simulink subsystem "MPC8_nlpsol"  (R2022b)
settings: Solver=VariableStepAuto  StartTime=0.0  StopTime=10.0  RelTol=1e-3
undefined symbols (not defined in the file): param_global, param_jointspace_ct, param_MPC8, param_robot, param_traj_data, param_weight_init
settings Model: Creator=emu  LastModifiedBy=emu
settings OptimizationCC: ReuseModelBlockBuffer=on

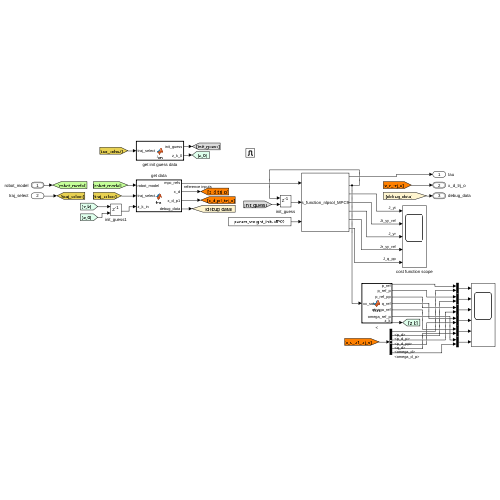
[thumbnail: Simulink's stored preview of the top-level diagram]
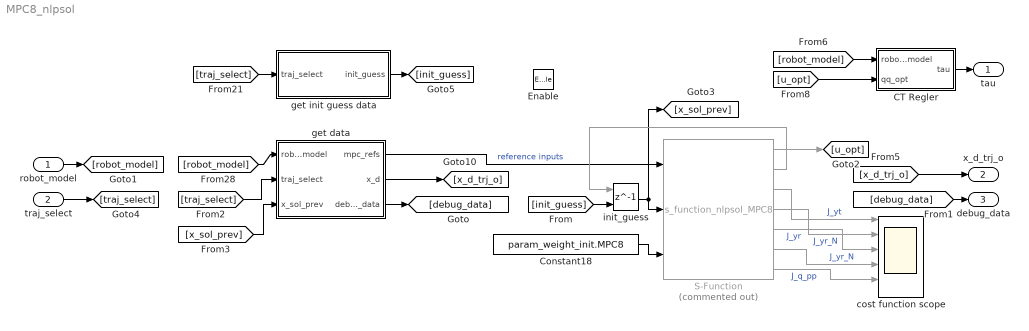
== system MPC8_nlpsol ==
  robot_model : Inport  OutDataTypeStr=Bus: robot_model
  traj_select : Inport  Port=2
  Enable : EnablePort
  CT Regler : MATLAB Function  TreatAsAtomicUnit=on
  Constant18 : Constant  Value=param_weight_init.MPC8  VectorParams1D=off
  S-Function : S-Function  Commented=on  FunctionName=s_function_nlpsol_MPC8  Parameters='s_functions/ur5e_6dof/MPC8.casadi', 'MPC8'  SFunctionModules='MPC8'  SFunctionDeploymentMode=off  EnableBusSupport=off
  cost function scope : Scope  NumInputPorts=6
  get data : MATLAB Function  TreatAsAtomicUnit=on
  get init guess data : MATLAB Function  TreatAsAtomicUnit=on
  init_guess : Delay  DelayLength=1  InitialConditionSource=Input port  InitialCondition=1
      settings: InputPortMap=u0,p4
  tau : Outport
  x_d_trj_o : Outport  Port=2  OutDataTypeStr=Bus: x_d
  debug_data : Outport  Port=3  OutDataTypeStr=Bus: debug_data_bus
  wires:
  S-Function/1 -> [u_opt]
  CT Regler/1(tau) -> tau/1
  [u_opt] -> CT Regler/2(qq_opt)
  [robot_model] -> CT Regler/1(robot_model)
  [x_d_trj_o] -> x_d_trj_o/1
  S-Function/3 -> cost function scope/1  "J_yt"
  robot_model/1 -> [robot_model]
  get data/2(x_d) -> [x_d_trj_o]
  S-Function/7 -> cost function scope/5  "J_q_pp"
  [traj_select] -> get init guess data/1(traj_select)
  get data/1(mpc_refs) -> S-Function/1  "reference inputs"
  [robot_model] -> get data/1(robot_model)
  get init guess data/1(init_guess) -> [init_guess]
  traj_select/1 -> [traj_select]
  init_guess/1 -> [x_sol_prev], S-Function/2
  [traj_select] -> get data/2(traj_select)
  [init_guess] -> init_guess/2
  S-Function/5 -> cost function scope/3  "J_yr"
  get data/3(debug_data) -> [debug_data]
  [debug_data] -> debug_data/1
  Constant18/1 -> S-Function/3
  S-Function/2 -> init_guess/1
  S-Function/4 -> cost function scope/2  "J_yr_N"
  S-Function/6 -> cost function scope/4  "J_yr_N"
  ? -> cost function scope/6  "J_du"
  [x_sol_prev] -> get data/3(x_sol_prev)

== matlab function MPC8_nlpsol/CT Regler ==
  data: robot_model input Bus: robot_model; tau output; qq_opt input; param_robot parameter; param_jointspace_ct parameter; param_global parameter
function tau = fcn(robot_model, qq_opt, param_robot, param_jointspace_ct, param_global)

n = param_robot.n_DOF;

if size(qq_opt, 2) ~= 0 && size(qq_opt, 1) ~= 1
    Ta = param_global.Ta;
    q = robot_model.q;      % generalized coordinates
    q_p = robot_model.q_p;  % time derivative of generalized coordinates
    
    q_d = qq_opt(1:n);
    q_d_p = qq_opt(n+1:2*n);
    q_d_pp = qq_opt(2*n+1:end);
    
    %q_d = q_d_0 + Ta*q_d_p_0;
    %q_d_p = q_d_p_0 + Ta*q_d_pp_0;
    %q_d_pp = q_d_pp_0;

    M = robot_model.M;      % inertia matrix
    C_rnea = robot_model.C_rnea; % C_rnea(q, q_p) = C(q, q_p)q_p + g(q) = n(q, q_p)
    
    e = q - q_d;
    e_p = q_p - q_d_p;
    
    K_D_q = param_jointspace_ct.MPC8.K_D_q;
    K_P_q = param_jointspace_ct.MPC8.K_P_q;
    tau = M*(q_d_pp - K_D_q * e_p - K_P_q * e) + C_rnea;
else
    tau = zeros(n,1);
end

== matlab function MPC8_nlpsol/get data ==
  settings: updateMethod=DISCRETE  sampleTime=param_global.Ta
  data: mpc_refs output; robot_model input Bus: robot_model; param_MPC8 parameter; x_d output Bus: x_d; debug_data output Bus: debug_data_bus; param_traj_data parameter; traj_select input; param_global parameter; x_sol_prev input
function [mpc_refs, x_d, debug_data] = fcn(robot_model, param_MPC8, param_traj_data, traj_select, param_global, x_sol_prev)
persistent cnt;

if(isempty(cnt))
    cnt = 1;
end

param_MPC = param_MPC8;
N         = param_MPC.N;
N_step    = param_MPC.N_step;
Ta = param_global.Ta;
u_indices = param_MPC.tau;
n = param_MPC.tau_dim(1);

% Parameters
q    = robot_model.q;      % generalized coordinates
q_p  = robot_model.q_p;  % time derivative of generalized coordinates
q_pp = robot_model.q_pp;
H    = robot_model.H;
J    = robot_model.J;
J_p  = robot_model.J_p;

R = H(1:3,1:3);% desired Orientation as rotational matrix
R_d = param_traj_data.R_d(:,:, cnt, traj_select);
q_d = param_traj_data.q_d(:, cnt, traj_select);

%y_q_err = quat_mult(y_q_e, quat_inv(param_traj_data.q_d(1:4, cnt, traj_select)));
q_err = rotm2quat_v4(R*R_d');
%y_q_e = rotm2quat_v4(R);
q_e = quat_mult(q_d, q_err);

% Current Pose of Endeffector
y = [H(1:3,4); q_e];
y_p = J*q_p;
y_pp = J*q_pp + J_p*q_p;

x_k = [q;q_p];

% Assemble vector of recieved output measurements
p_d     = param_traj_data.p_d(   1:3, cnt : N_step : cnt + (N)*N_step, traj_select);
q_d     = param_traj_data.q_d(   1:4, cnt : N_step : cnt + (N)*N_step, traj_select);

omega_d   = param_traj_data.omega_d(  1:3, cnt : N_step : cnt + (N)*N_step, traj_select);
omega_d_p = param_traj_data.omega_d_p(1:3, cnt : N_step : cnt + (N)*N_step, traj_select);

alpha_d    = param_traj_data.alpha_d(           :, cnt : N_step : cnt + (N)*N_step, traj_select);
alpha_d_p  = param_traj_data.alpha_d_p(         :, cnt : N_step : cnt + (N)*N_step, traj_select);
alpha_d_pp = param_traj_data.alpha_d_pp(        :, cnt : N_step : cnt + (N)*N_step, traj_select);
rot_ax_d   = param_traj_data.rot_ax_d(          :, cnt : N_step : cnt + (N)*N_step, traj_select);
alpha_d_offset = param_traj_data.alpha_d_offset(:, cnt : N_step : cnt + (N)*N_step, traj_select);
q_d_rel = param_traj_data.q_d_rel(              :, cnt : N_step : cnt + (N)*N_step, traj_select);

kin_int_mode = struct;
kin_int_mode.standard = 1;
kin_int_mode.du0_cost = 2;
kin_int_mode.du_cost_extended = 3;

mpc_mode = kin_int_mode.standard;

if(mpc_mode == kin_int_mode.standard || mpc_mode == kin_int_mode.du0_cost)
    p_d_kp1 = param_traj_data.p_d(   1:3, cnt+1, traj_select);
    q_d_kp1 = param_traj_data.q_d(   1:4, cnt+1, traj_select);
    if(N_step == 1)
        y_d = [p_d; q_d];
    else
        y_d    = [[p_d(:,1), p_d_kp1, p_d(:,2:end-1)]; [q_d(:,1), q_d_kp1, q_d(:,2:end-1)]];
    end
else %if(mpc_mode == kin_int_mode.du_cost_extended)
    % N must be odd!
    p_d_kp1 = param_traj_data.p_d(   1:3, cnt+1 : N_step : cnt+1 + (N)*N_step, traj_select);
    q_d_kp1 = param_traj_data.q_d(   1:4, cnt+1 : N_step : cnt+1 + (N)*N_step, traj_select);

    N2 = round((N+1)/2);

    y_d_k = [p_d(:, 1:1:N2); q_d(:, 1:1:N2)];
    y_d_kp1 = [p_d_kp1(:, 1:1:N2); q_d_kp1(:, 1:1:N2)];

    y_d = reshape([y_d_k; y_d_kp1], 7, N+1);
end



%% Reference out
if(mpc_mode == kin_int_mode.standard)
    mpc_refs = [x_k(:); y_d(:)];
elseif(mpc_mode == kin_int_mode.du0_cost)
    u_prev = x_sol_prev(u_indices(n+1:2*n));
    mpc_refs = [x_k(:); y_d(:); u_prev(:)];
else %if(mpc_mode == kin_int_mode.du_cost_extended)
    u_prev_indices = (1:n)' .*(ones(n,1)) + (n:2*n:n*(N-1));
    u_prev = x_sol_prev(u_indices(u_prev_indices(:)));
    mpc_refs = [x_k(:); y_d(:); u_prev(:)];
end


%% TRAJECTORY OUT
x_d.p_d       = param_traj_data.p_d(1:3, cnt , traj_select);    %y0
x_d.p_d_p     = param_traj_data.p_d_p(1:3, cnt , traj_select);  %y0p
x_d.p_d_pp    = param_traj_data.p_d_pp(1:3, cnt , traj_select); %y0pp
x_d.Phi_d     = param_traj_data.Phi_d(:, cnt , traj_select);
x_d.Phi_d_p   = param_traj_data.Phi_d_p(:, cnt, traj_select);
x_d.Phi_d_pp  = param_traj_data.Phi_d_pp(:,cnt, traj_select);
x_d.R_d       = R_d;
x_d.q_d       = q_d(1:4, 1);
x_d.q_d_p     = param_traj_data.q_d_p(1:4, cnt, traj_select);
x_d.q_d_pp    = param_traj_data.q_d_pp(1:4, cnt, traj_select);
x_d.omega_d   = omega_d(1:3, 1);
x_d.omega_d_p = omega_d_p(1:3, 1);
x_d.alpha_d    = alpha_d(:, 1);
x_d.alpha_d_p  = alpha_d_p(:, 1);
x_d.alpha_d_pp = alpha_d_pp(:, 1);
x_d.rot_ax_d   = rot_ax_d(:, 1);
x_d.alpha_d_offset = alpha_d_offset(:, 1);
x_d.q_d_rel = q_d_rel(:, 1);

%% DEBUG
debug_data.p           = y(1:3);
debug_data.p_p         = y_p(1:3);
debug_data.p_pp        = y_pp(1:3);
debug_data.Phi     = rotm2eul_v2(R);
debug_data.Phi_p   = [0; 0; 0]; % ?????? Phi_p = T * omega?
debug_data.Phi_pp  = [0; 0; 0]; % ??????
debug_data.q           = y(4:7);
debug_data.omega       = y_p(4:6);
debug_data.omega_p     = y_pp(4:6);
debug_data.p_err       = y(1:3) - param_traj_data.p_d(:, cnt, traj_select);
debug_data.p_p_err     = y_p(1:3) - param_traj_data.p_d_p(:, cnt, traj_select);
debug_data.p_pp_err    = y_pp(1:3) - param_traj_data.p_d_pp(:, cnt, traj_select);
debug_data.q_err       = q_err;
debug_data.omega_err   = y_p(4:6)  - omega_d(1:3, 1);
debug_data.omega_p_err = y_pp(4:6) - omega_d_p(1:3, 1);

cnt = cnt+1;

== matlab function MPC8_nlpsol/get init guess data ==
  data: traj_select input; param_MPC8_init_guess parameter; init_guess output
function init_guess   = fcn(traj_select, param_MPC8_init_guess)

%init_guess = param_MPC8_init_guess.init_guess(1,:);
init_guess = param_MPC8_init_guess.init_guess(traj_select,:);
